simulink model "RealEstado1"  (R2023b)
settings: Solver=VariableStepAuto  StartTime=0.0  StopTime=10.0  RelTol=1e-3
settings Model: Creator=User  LastModifiedBy=User

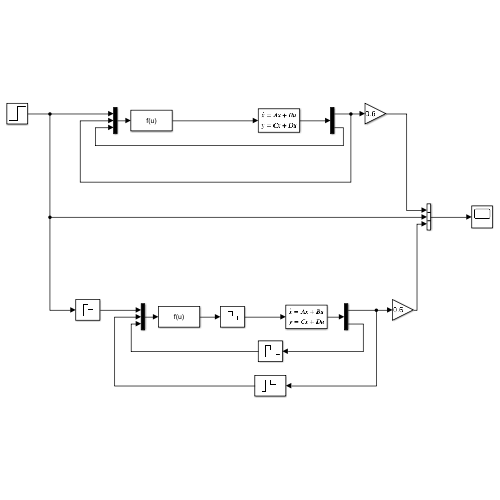
[thumbnail: Simulink's stored preview of the top-level diagram]
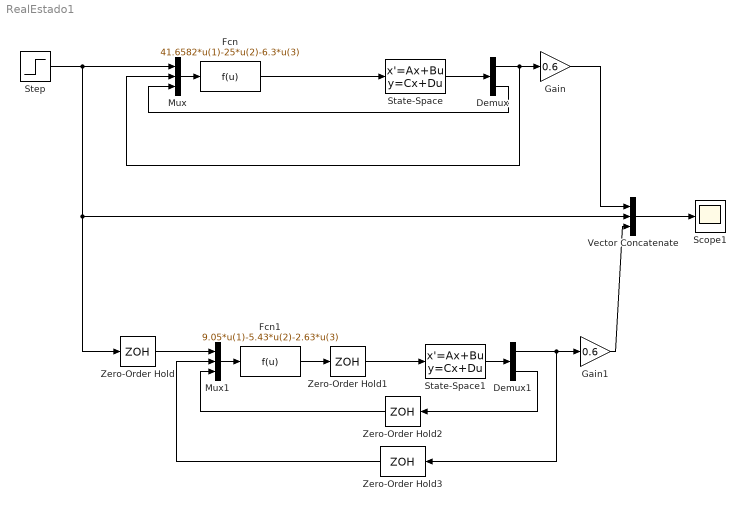
== system RealEstado1 ==
  Demux : Demux  Outputs=2
  Demux1 : Demux  Outputs=2
  Fcn : Fcn  Expr=41.6582*u(1)-25*u(2)-6.3*u(3)
  Fcn1 : Fcn  Expr=9.05*u(1)-5.43*u(2)-2.63*u(3)
  Gain : Gain  Gain=0.6
  Gain1 : Gain  Gain=0.6
  Mux : Mux  Inputs=3
  Mux1 : Mux  Inputs=3
  Scope1 : Scope
  State-Space : StateSpace  A=[0 1; 0 -0.7]  B=[0; 1]  C=eye(2)  D=[0;0]  InitialCondition=0
  State-Space1 : StateSpace  A=[0 1; 0 -0.7]  B=[0; 1]  C=eye(2)  D=[0;0]  InitialCondition=0
  Step : Step  SampleTime=0
  Vector Concatenate : Concatenate  NumInputs=3
  Zero-Order Hold{,1..3} (4 alike) : ZeroOrderHold  SampleTime=0.05
  wires:
  Mux/1 -> Fcn/1
  Demux/2 -> Mux/3
  State-Space/1 -> Demux/1
  Fcn/1 -> State-Space/1
  Step/1 -> Vector Concatenate/2, Zero-Order Hold/1, Mux/1
  Demux/1 -> Gain/1, Mux/2
  Mux1/1 -> Fcn1/1
  Gain1/1 -> Vector Concatenate/3
  State-Space1/1 -> Demux1/1
  Demux1/1 -> Zero-Order Hold3/1, Gain1/1
  Zero-Order Hold/1 -> Mux1/1
  Fcn1/1 -> Zero-Order Hold1/1
  Zero-Order Hold1/1 -> State-Space1/1
  Demux1/2 -> Zero-Order Hold2/1
  Zero-Order Hold2/1 -> Mux1/3
  Zero-Order Hold3/1 -> Mux1/2
  Gain/1 -> Vector Concatenate/1
  Vector Concatenate/1 -> Scope1/1
